simulink model "comparison"  (Simulink 7.6)
settings: Solver=ode45  StartTime=0.0  StopTime=10  RelTol=1e-3
libraries: simulink x14
settings Model: Creator=Docencia  LastModifiedBy=Docencia

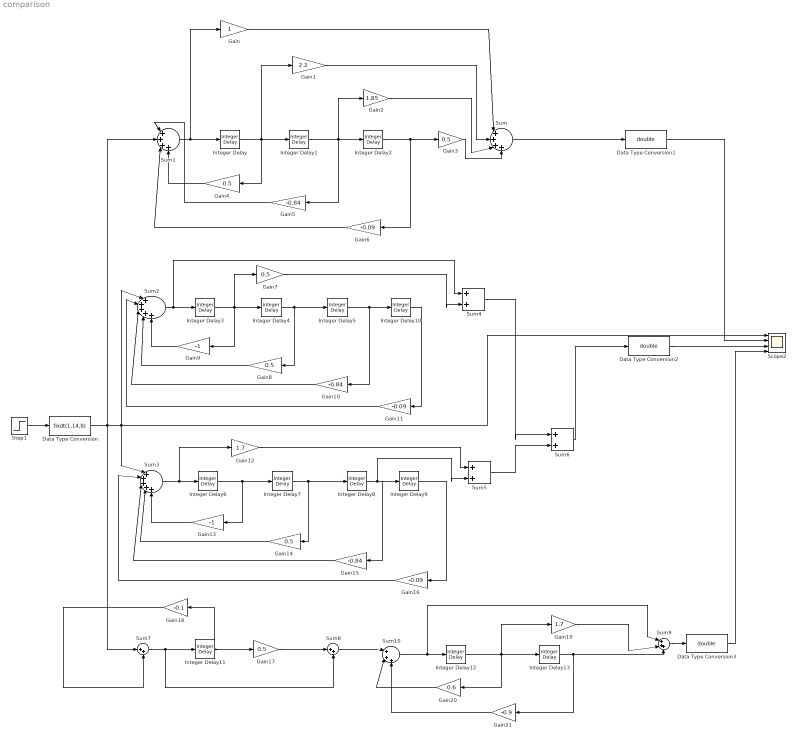
== system comparison ==
  Data Type Conversion : DataTypeConversion  OutDataTypeStr=fixdt(1,14,8)  SaturateOnIntegerOverflow=on
  Data Type Conversion1 : DataTypeConversion  OutDataTypeStr=double
  Data Type Conversion2 : DataTypeConversion  OutDataTypeStr=double
  Data Type Conversion3 : DataTypeConversion  OutDataTypeStr=double
  Gain : Gain  ParamDataTypeStr=sfix(8)  OutDataTypeStr=fixdt(1,14,8)
  Gain1 : Gain  Gain=2.2  ParamDataTypeStr=sfix(8)  OutDataTypeStr=fixdt(1,14,8)
  Gain10 : Gain  Gain=-0.84  ParamDataTypeStr=sfix(8)  OutDataTypeStr=fixdt(1,14,8)
  Gain11 : Gain  Gain=-0.09  ParamDataTypeStr=sfix(8)  OutDataTypeStr=fixdt(1,14,8)
  Gain12 : Gain  Gain=1.7  ParamDataTypeStr=sfix(8)  OutDataTypeStr=fixdt(1,14,8)
  Gain13 : Gain  Gain=-1  ParamDataTypeStr=sfix(8)  OutDataTypeStr=fixdt(1,14,8)
  Gain{3..4,7..8,14,17} (6 alike) : Gain  Gain=0.5  ParamDataTypeStr=sfix(8)  OutDataTypeStr=fixdt(1,14,8)
  Gain15 : Gain  Gain=-0.84  ParamDataTypeStr=sfix(8)  OutDataTypeStr=fixdt(1,14,8)
  Gain16 : Gain  Gain=-0.09  ParamDataTypeStr=sfix(8)  OutDataTypeStr=fixdt(1,14,8)
  Gain18 : Gain  Gain=-0.1  ParamDataTypeStr=sfix(8)  OutDataTypeStr=fixdt(1,14,8)
  Gain19 : Gain  Gain=1.7  ParamDataTypeStr=sfix(8)  OutDataTypeStr=fixdt(1,14,8)
  Gain2 : Gain  Gain=1.85  ParamDataTypeStr=sfix(8)  OutDataTypeStr=fixdt(1,14,8)
  Gain20 : Gain  Gain=0.6  ParamDataTypeStr=sfix(8)  OutDataTypeStr=fixdt(1,14,8)
  Gain21 : Gain  Gain=-0.9  ParamDataTypeStr=sfix(8)  OutDataTypeStr=fixdt(1,14,8)
  Gain5 : Gain  Gain=-0.84  ParamDataTypeStr=sfix(8)  OutDataTypeStr=fixdt(1,14,8)
  Gain6 : Gain  Gain=-0.09  ParamDataTypeStr=sfix(8)  OutDataTypeStr=fixdt(1,14,8)
  Gain9 : Gain  Gain=-1  ParamDataTypeStr=sfix(8)  OutDataTypeStr=fixdt(1,14,8)
  Integer Delay{,1..13} (14 alike) : simulink/Discrete/Integer Delay  NumDelays=1  vinit=0.0  samptime=-1
  Scope2 : Scope  NumInputPorts=4
      settings: YMin=-5~-5~-5~-5  YMax=5~5~5~5  SaveName=ScopeData2
  Step1 : Step  Time=2  SampleTime=0
  Sum : Sum  Inputs=|++++
  Sum1 : Sum  Inputs=|++++
  Sum10 : Sum  Inputs=|+++
  Sum2 : Sum  Inputs=|+++++
  Sum3 : Sum  Inputs=|+++++
  Sum{4..8} (5 alike) : Sum  Inputs=|++
  Sum9 : Sum  Inputs=|+++
  wires:
  Integer Delay/1 -> Integer Delay1/1, Gain1/1, Gain4/1
  Integer Delay1/1 -> Integer Delay2/1, Gain2/1, Gain5/1
  Integer Delay2/1 -> Gain3/1, Gain6/1
  Gain/1 -> Sum/1
  Gain1/1 -> Sum/2
  Gain2/1 -> Sum/3
  Gain3/1 -> Sum/4
  Sum1/1 -> Integer Delay/1, Gain/1
  Gain6/1 -> Sum1/3
  Gain5/1 -> Sum1/1
  Gain4/1 -> Sum1/4
  Step1/1 -> Data Type Conversion/1
  Sum2/1 -> Integer Delay3/1, Sum4/1
  Integer Delay3/1 -> Integer Delay4/1, Gain7/1, Gain9/1
  Integer Delay4/1 -> Integer Delay5/1, Gain8/1
  Gain7/1 -> Sum4/2
  Integer Delay5/1 -> Integer Delay10/1, Gain10/1
  Integer Delay10/1 -> Gain11/1
  Gain11/1 -> Sum2/2
  Gain10/1 -> Sum2/3
  Gain8/1 -> Sum2/4
  Gain9/1 -> Sum2/5
  Sum3/1 -> Integer Delay6/1, Gain12/1
  Integer Delay6/1 -> Integer Delay7/1, Gain13/1
  Integer Delay7/1 -> Integer Delay8/1, Gain14/1
  Gain12/1 -> Sum5/1
  Integer Delay8/1 -> Sum5/2, Integer Delay9/1, Gain15/1
  Integer Delay9/1 -> Gain16/1
  Gain16/1 -> Sum3/2
  Gain15/1 -> Sum3/3
  Gain14/1 -> Sum3/4
  Gain13/1 -> Sum3/5
  Sum4/1 -> Sum6/1
  Sum5/1 -> Sum6/2
  Sum7/1 -> Integer Delay11/1, Sum8/2
  Integer Delay11/1 -> Gain17/1, Gain18/1
  Gain17/1 -> Sum8/1
  Gain18/1 -> Sum7/2
  Integer Delay12/1 -> Gain19/1, Integer Delay13/1, Gain20/1
  Sum10/1 -> Integer Delay12/1, Sum9/1
  Integer Delay13/1 -> Gain21/1, Sum9/3
  Gain19/1 -> Sum9/2
  Gain20/1 -> Sum10/2
  Gain21/1 -> Sum10/3
  Sum8/1 -> Sum10/1
  Sum/1 -> Data Type Conversion1/1
  Sum6/1 -> Data Type Conversion2/1
  Sum9/1 -> Data Type Conversion3/1
  Data Type Conversion1/1 -> Scope2/2
  Data Type Conversion2/1 -> Scope2/3
  Data Type Conversion3/1 -> Scope2/4
  Data Type Conversion/1 -> Sum2/1, Sum3/1, Scope2/1, Sum1/2, Sum7/1
